simulink model "C1_Calculation"  (R2024a)
settings: Solver=VariableStepAuto  StartTime=0.0  StopTime=10.0  RelTol=1e-3
settings Model: Creator=ACER  LastModifiedBy=ACER

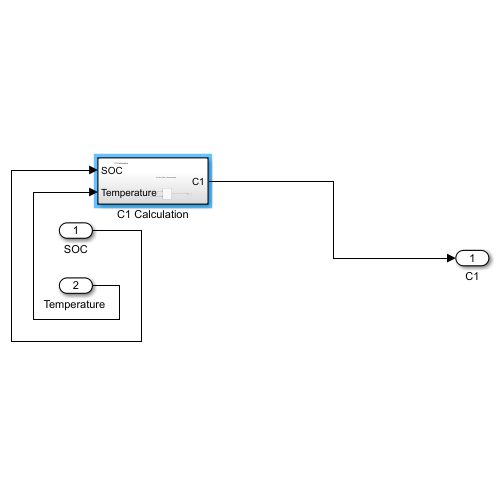
[thumbnail: Simulink's stored preview of the top-level diagram]
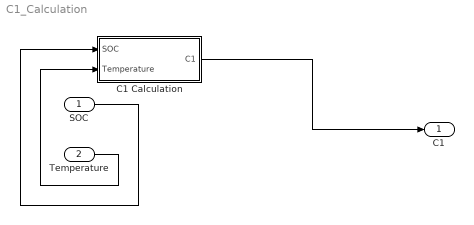
== system C1_Calculation ==
  SOC : Inport
  "Temperature " : Inport  Port=2
  C1 Calculation : Subsystem
  C1 : Outport
  wires:
  SOC/1 -> C1 Calculation/1(SOC)
  "Temperature "/1 -> C1 Calculation/2("Temperature ")
  C1 Calculation/1(C1) -> C1/1

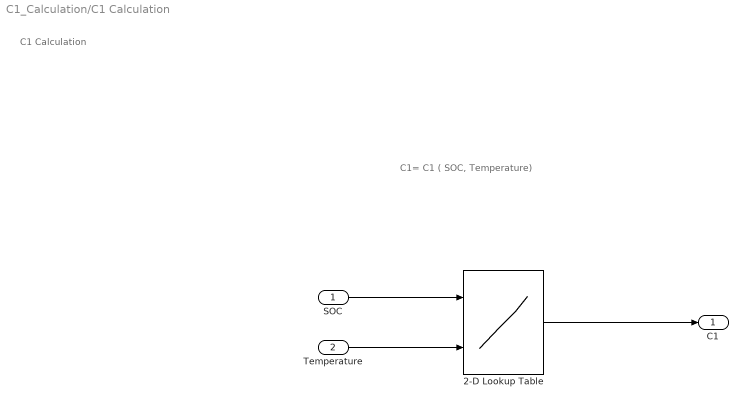
== system C1_Calculation/C1 Calculation ==
  note: C1 Calculation
  note: C1= C1 ( SOC, Temperature)
  SOC : Inport
  "Temperature " : Inport  Port=2
  2-D Lookup Table : Lookup_n-D  BreakpointsForDimension1=[1:3]  BreakpointsForDimension2=[1:3]  InternalRulePriority=Speed  RndMeth=Simplest
      settings: InputPortMap=u0,u1
  C1 : Outport
  wires:
  2-D Lookup Table/1 -> C1/1
  SOC/1 -> 2-D Lookup Table/1
  "Temperature "/1 -> 2-D Lookup Table/2
